simulink model "LogicalConditioning"  (R2024a)
settings: Solver=VariableStepAuto  StartTime=0.0  StopTime=100  MaxStep=0.01  RelTol=1e-3
settings Model: Creator=ammaa  LastModifiedBy=ammaa

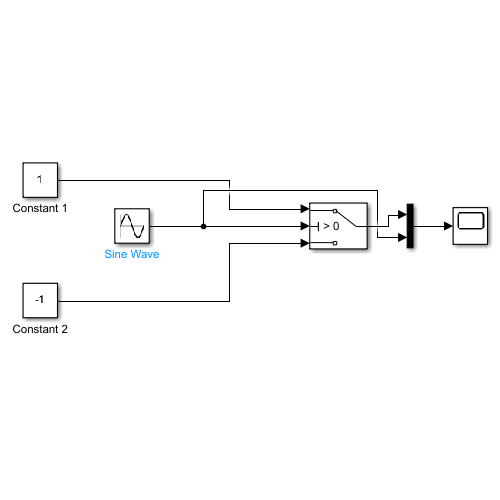
[thumbnail: Simulink's stored preview of the top-level diagram]
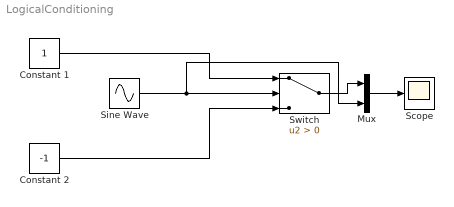
== system LogicalConditioning ==
  Constant 1 : Constant
  Constant 2 : Constant  Value=-1
  Mux : Mux  Inputs=2
  Scope : Scope
  Sine Wave : Sin  SampleTime=0
  Switch : Switch  Criteria=u2 > Threshold  SaturateOnIntegerOverflow=off  InputSameDT=off
  wires:
  Constant 1/1 -> Switch/1
  Constant 2/1 -> Switch/3
  Switch/1 -> Mux/1
  Sine Wave/1 -> Mux/2, Switch/2
  Mux/1 -> Scope/1
